simulink model "CAN_Model_v2"  (R2018b)
settings: Solver=VariableStepAuto  StartTime=0.0  StopTime=20  RelTol=1e-3
libraries: simulink_extras x1
settings Model: Creator=Emiliano  LastModifiedBy=Emiliano

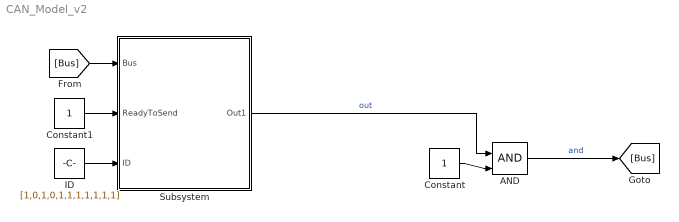
== system CAN_Model_v2 ==
  AND : Logic  IconShape=distinctive  AllPortsSameDT=off  OutDataTypeStr=boolean
  Constant : Constant  SampleTime=0.2
  Constant1 : Constant
  ID : Constant  Value=[1,0,1,0,1,1,1,1,1,1,1]
  Subsystem : Subsystem
  wires:
  Subsystem/1(Out1) -> AND/1  "out"
  Constant/1 -> AND/2
  AND/1 -> [Bus]  "and"
  [Bus] -> Subsystem/1(Bus)
  Constant1/1 -> Subsystem/2("ReadyToSend ")
  ID/1 -> Subsystem/3(ID)

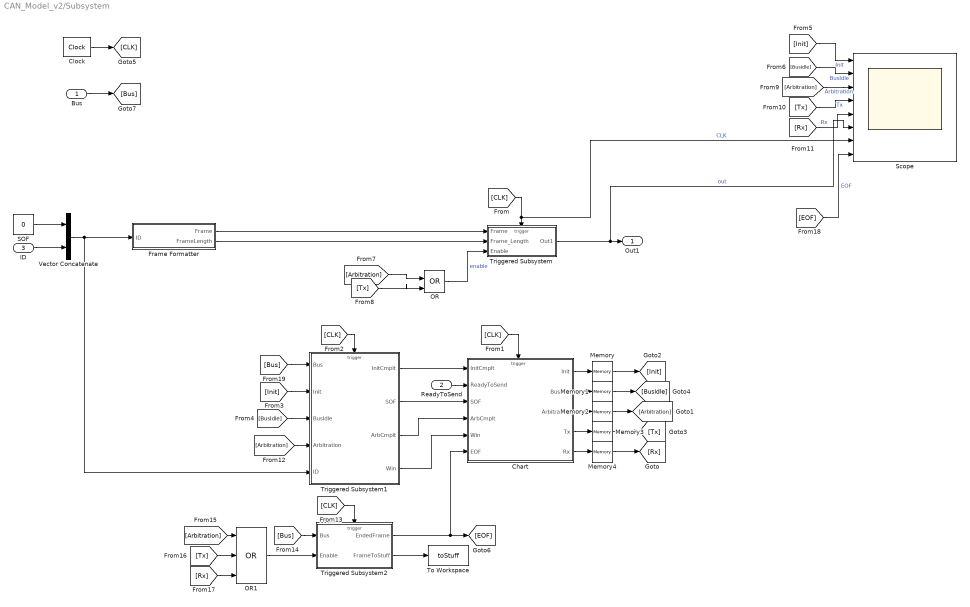
== system CAN_Model_v2/Subsystem ==
  Bus : Inport
  "ReadyToSend " : Inport  Port=2
  ID : Inport  Port=3
  Chart : Stateflow chart  TreatAsAtomicUnit=on
  Clock : simulink_extras/Flip Flops/Clock  period=0.2
  Frame Formatter : Subsystem
  Memory{,1..4} (5 alike) : Memory
  OR : Logic  Operator=OR  IconShape=distinctive  AllPortsSameDT=off  OutDataTypeStr=boolean
  OR1 : Logic  Operator=OR  Inputs=3  IconShape=distinctive  AllPortsSameDT=off  OutDataTypeStr=boolean
  SOF : Constant  Value=0
  Scope : Scope  NumInputPorts=8
  To Workspace : ToWorkspace  VariableName=toStuff  SaveFormat=Timeseries  SampleTime=-1
  Triggered Subsystem : Subsystem  TreatAsAtomicUnit=on
  Triggered Subsystem1 : Subsystem  TreatAsAtomicUnit=on
  Triggered Subsystem2 : Subsystem  TreatAsAtomicUnit=on
  Vector Concatenate : Concatenate
  Out1 : Outport
  wires:
  [CLK] -> Chart/Trigger
  [Arbitration] -> OR/1
  [Tx] -> OR/2
  OR/1 -> Triggered Subsystem/3(Enable)  "enable"
  Chart/5(" Rx") -> Memory4/1
  Chart/3(" Arbitration") -> Memory2/1
  Chart/1(" Init") -> Memory/1
  Chart/4(" Tx") -> Memory3/1
  Chart/2(" BusIdle") -> Memory1/1
  Clock/1 -> [CLK]
  [CLK] -> Scope/7, Triggered Subsystem/Trigger  "CLK"
  [CLK] -> Triggered Subsystem1/Trigger
  Triggered Subsystem1/1(InitCmplt) -> Chart/1(InitCmplt)
  [Init] -> Triggered Subsystem1/2(Init)
  "ReadyToSend "/1 -> Chart/2(ReadyToSend)
  [BusIdle] -> Triggered Subsystem1/3(BusIdle)
  Triggered Subsystem1/2(SOF) -> Chart/3(SOF)
  Triggered Subsystem1/4(Win) -> Chart/5(Win)
  Triggered Subsystem1/3("ArbCmplt ") -> Chart/4(ArbCmplt)
  [Init] -> Scope/1  "Init"
  [BusIdle] -> Scope/2  "BusIdle"
  [Arbitration] -> Scope/3  "Arbitration"
  [Tx] -> Scope/4  "Tx"
  [Rx] -> Scope/5  "Rx"
  Memory/1 -> [Init]
  Memory1/1 -> [BusIdle]
  Memory2/1 -> [Arbitration]
  Memory3/1 -> [Tx]
  Memory4/1 -> [Rx]
  Triggered Subsystem/1(Out1) -> Scope/6, Out1/1  "out"
  ID/1 -> Vector Concatenate/2
  [Arbitration] -> Triggered Subsystem1/4(Arbitration)
  [CLK] -> Triggered Subsystem2/Trigger
  [Bus] -> Triggered Subsystem2/1(Bus)
  OR1/1 -> Triggered Subsystem2/2(Enable)
  [Arbitration] -> OR1/1
  [Tx] -> OR1/2
  [Rx] -> OR1/3
  Triggered Subsystem2/1(EndedFrame) -> [EOF], Chart/6(EOF)
  Triggered Subsystem2/2(FrameToStuff) -> To Workspace/1
  [EOF] -> Scope/8  "EOF"
  Bus/1 -> [Bus]
  [Bus] -> Triggered Subsystem1/1(Bus)
  SOF/1 -> Vector Concatenate/1
  Vector Concatenate/1 -> Triggered Subsystem1/5(ID), Frame Formatter/1(ID)
  Frame Formatter/1(Frame) -> Triggered Subsystem/1("Frame ")
  Frame Formatter/2("FrameLength ") -> Triggered Subsystem/2(Frame_Length)

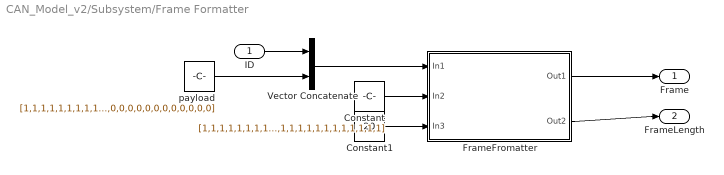
== system CAN_Model_v2/Subsystem/Frame Formatter ==
  ID : Inport
  Constant : Constant  Value=[1,1,1,1,1,1,1,1,1,1,1,1,1,1,1,1,1,1,1,1]
  Constant1 : Constant  Value=20
  FrameFromatter : Subsystem
  Vector Concatenate : Concatenate
  "payload " : Constant  Value=[1,1,1,1,1,1,1,1,1,1,1,1,1,1,1,1,1,1,1,0,0,0,0,0,0,0,0,0,0,0,0,0,0,0,0,0]
  Frame : Outport
  "FrameLength " : Outport  Port=2
  wires:
  ID/1 -> Vector Concatenate/1
  "payload "/1 -> Vector Concatenate/2
  Vector Concatenate/1 -> FrameFromatter/1(In1)
  Constant/1 -> FrameFromatter/2(In2)
  Constant1/1 -> FrameFromatter/3(In3)
  FrameFromatter/1(Out1) -> Frame/1
  FrameFromatter/2(Out2) -> "FrameLength "/1

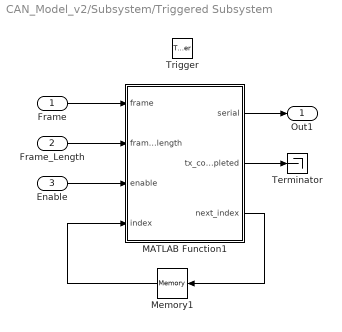
== system CAN_Model_v2/Subsystem/Triggered Subsystem ==
  "Frame " : Inport
  Frame_Length : Inport  Port=2
  Enable : Inport  Port=3
  Trigger : TriggerPort  VariantControl=Variant
  MATLAB Function1 : MATLAB Function  TreatAsAtomicUnit=on
  Memory1 : Memory  InitialCondition=1  InheritSampleTime=on
  Terminator : Terminator
  Out1 : Outport
  wires:
  Memory1/1 -> MATLAB Function1/4(index)
  MATLAB Function1/1(serial) -> Out1/1
  MATLAB Function1/3(next_index) -> Memory1/1
  MATLAB Function1/2(tx_completed) -> Terminator/1
  Enable/1 -> MATLAB Function1/3(enable)
  "Frame "/1 -> MATLAB Function1/1(frame)
  Frame_Length/1 -> MATLAB Function1/2(frame_length)

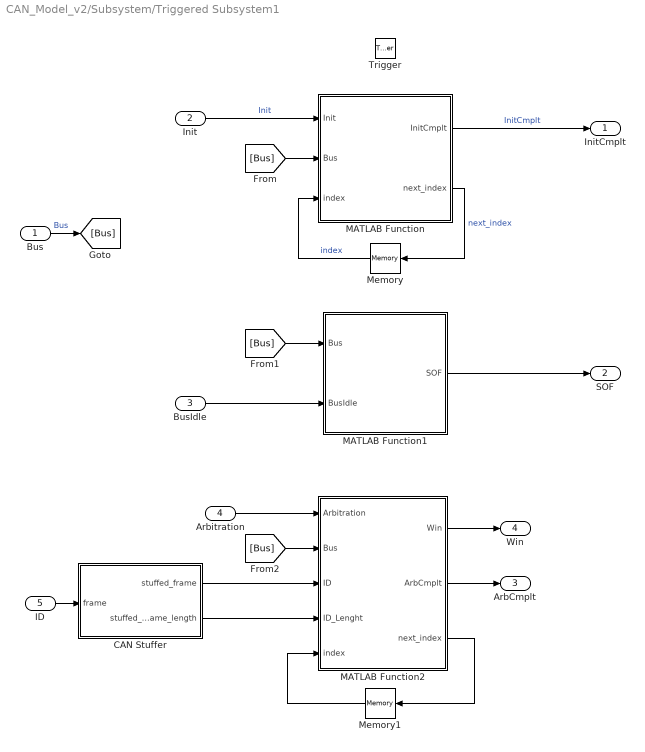
== system CAN_Model_v2/Subsystem/Triggered Subsystem1 ==
  Bus : Inport
  Init : Inport  Port=2
  BusIdle : Inport  Port=3
  Arbitration : Inport  Port=4
  ID : Inport  Port=5
  Trigger : TriggerPort  VariantControl=Variant
  CAN Stuffer : MATLAB Function  TreatAsAtomicUnit=on
  MATLAB Function : MATLAB Function  TreatAsAtomicUnit=on
  MATLAB Function1 : MATLAB Function  TreatAsAtomicUnit=on
  MATLAB Function2 : MATLAB Function  TreatAsAtomicUnit=on
  Memory : Memory  InheritSampleTime=on
  Memory1 : Memory  InitialCondition=1  InheritSampleTime=on
  InitCmplt : Outport
  SOF : Outport  Port=2
  "ArbCmplt " : Outport  Port=3
  Win : Outport  Port=4
  wires:
  MATLAB Function/2(next_index) -> Memory/1  "next_index"
  Memory/1 -> MATLAB Function/3(index)  "index"
  MATLAB Function/1(InitCmplt) -> InitCmplt/1  "InitCmplt"
  MATLAB Function1/1(SOF) -> SOF/1
  Init/1 -> MATLAB Function/1(Init)  "Init"
  BusIdle/1 -> MATLAB Function1/2(BusIdle)
  Arbitration/1 -> MATLAB Function2/1(Arbitration)
  Bus/1 -> [Bus]  "Bus"
  [Bus] -> MATLAB Function/2(Bus)
  [Bus] -> MATLAB Function1/1(Bus)
  [Bus] -> MATLAB Function2/2(Bus)
  MATLAB Function2/3(next_index) -> Memory1/1
  Memory1/1 -> MATLAB Function2/5(index)
  MATLAB Function2/1(Win) -> Win/1
  MATLAB Function2/2(ArbCmplt) -> "ArbCmplt "/1
  ID/1 -> CAN Stuffer/1(frame)
  CAN Stuffer/1(stuffed_frame) -> MATLAB Function2/3(ID)
  CAN Stuffer/2(stuffed_frame_length) -> MATLAB Function2/4(ID_Lenght)

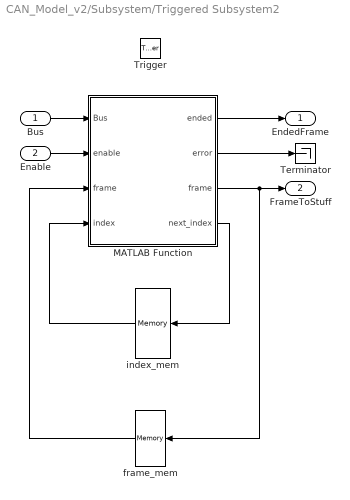
== system CAN_Model_v2/Subsystem/Triggered Subsystem2 ==
  Bus : Inport
  Enable : Inport  Port=2
  Trigger : TriggerPort  VariantControl=Variant
  MATLAB Function : MATLAB Function  TreatAsAtomicUnit=on
  Terminator : Terminator
  frame_mem : Memory  InitialCondition=[0,0,0,0,0,0,0,0,0,0,0,0,0,0,0,0,0,0,0,0,0,0,0,0,0,0,0,0,0,0,0,0,0,0,0,0,0,0,0,0,0,0,0,0,0,0,0,0,0,0,0,0,0,0,0,0,0,0,0,0,0,0,0,0,0,0,0,0,0,0,0,0,0,0,0,0,0,0,0,0,0,0,0,0,0,0,0,0,0,0,0,0,0,0,0,0,0,0,0,0,0,0,0,0,0,0,0,0,0,0,0,0,0,0,0,0,0,0,0,0,0,0,0,0,0,0,0,0,0,0,0,0,0,0,0]  InheritSampleTime=on
  index_mem : Memory  InitialCondition=1  InheritSampleTime=on
  EndedFrame : Outport
  FrameToStuff : Outport  Port=2
  wires:
  Enable/1 -> MATLAB Function/2(enable)
  Bus/1 -> MATLAB Function/1(Bus)
  MATLAB Function/4(next_index) -> index_mem/1
  frame_mem/1 -> MATLAB Function/3("frame ")
  MATLAB Function/1(ended) -> EndedFrame/1
  MATLAB Function/3(frame) -> frame_mem/1, FrameToStuff/1
  index_mem/1 -> MATLAB Function/4(index)
  MATLAB Function/2(error) -> Terminator/1

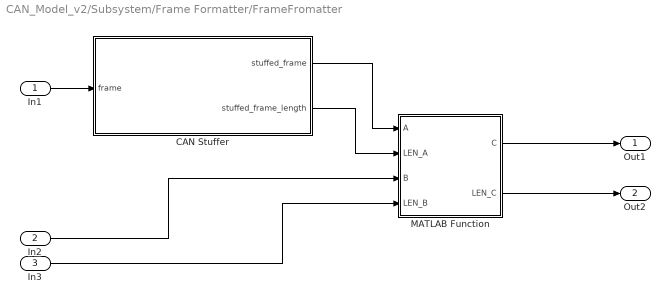
== system CAN_Model_v2/Subsystem/Frame Formatter/FrameFromatter ==
  In1 : Inport
  In2 : Inport  Port=2
  In3 : Inport  Port=3
  CAN Stuffer : MATLAB Function  TreatAsAtomicUnit=on
  MATLAB Function : MATLAB Function  TreatAsAtomicUnit=on
  Out1 : Outport
  Out2 : Outport  Port=2
  wires:
  MATLAB Function/2(LEN_C) -> Out2/1
  In1/1 -> CAN Stuffer/1(frame)
  CAN Stuffer/2(stuffed_frame_length) -> MATLAB Function/2(LEN_A)
  MATLAB Function/1(C) -> Out1/1
  In3/1 -> MATLAB Function/4(LEN_B)
  CAN Stuffer/1(stuffed_frame) -> MATLAB Function/1(A)
  In2/1 -> MATLAB Function/3(B)

== matlab function CAN_Model_v2/Subsystem/Triggered Subsystem1/MATLAB Function ==
  data: Init input; InitCmplt output; Bus input; index input; next_index output
function [InitCmplt, next_index] = BusIdleSensing(Init, Bus, index)

InitCmplt = 0;

if Init == 1
    if Bus == 1
        if index < 10 %Number of one to wait for EOF (after 11 ones)
            next_index = index + 1;
        else
            next_index = 0;
            InitCmplt = 1;
        end
    else
        next_index = 0;
    end
else
   next_index = 0;
end

end

== matlab function CAN_Model_v2/Subsystem/Triggered Subsystem/MATLAB Function1 ==
  data: frame input; frame_length input; enable input; serial output; tx_completed output; index input; next_index output
function [serial,  tx_completed ,next_index]  = fcn(frame, frame_length, enable, index)

if enable == 1
    if index > frame_length
        serial = 1;
        tx_completed = 1;
        next_index = 1;
    else
        serial = frame(index);
        next_index = index + 1;
        tx_completed = 0;
    end
else
    tx_completed = 0;
    serial = 1;
    next_index = 1;
end

end

== stateflow chart CAN_Model_v2/Subsystem/Chart ==
  settings: sampleTime=0.2  executeAtInitialization=1
  state Init
  state Rx
  state BusIdle
  state Arbitration
  state Tx
  Init -> Init [order 2] : [InitCmplt == 0]
  (default) -> Init
  Init -> BusIdle [order 1] : [InitCmplt == 1]
  Rx -> Rx [order 2] : [EOF == 0]
  BusIdle -> Rx [order 2] : [ReadyToSend == 0 && SOF == 1]
  Rx -> BusIdle [order 1] : [EOF == 1]
  BusIdle -> BusIdle [order 3] : [ReadyToSend == 0 && SOF == 0]
  Arbitration -> Rx [order 1] : [ArbCmplt ==1 && Win == 0]
  Tx -> BusIdle [order 2] : [EOF == 1]
  BusIdle -> Arbitration [order 1] : [ReadyToSend > 0]
  Arbitration -> Tx [order 2] : [ArbCmplt ==1 && Win == 1]
  Arbitration -> Arbitration [order 3] : [ArbCmplt == 0]
  Tx -> Tx [order 1] : [EOF == 0]
  data: Init output boolean; BusIdle output boolean; Arbitration output boolean; Tx output boolean; Rx output boolean; InitCmplt input; ReadyToSend input; SOF input; ArbCmplt input; Win input; EOF input
  events: Start input FALLING_EDGE_EVENT

== matlab function CAN_Model_v2/Subsystem/Triggered Subsystem1/MATLAB Function1 ==
  data: Bus input; SOF output; BusIdle input
function SOF = SOF_Detection(Bus, BusIdle)

if BusIdle == 1 %Checks the current state of the FSM
    if Bus == 0
        SOF = 1; %SOF Detected, the flag goes to One!
    else
        SOF = 0;    
    end
else
    SOF = 0;
end

end

== matlab function CAN_Model_v2/Subsystem/Triggered Subsystem1/MATLAB Function2 ==
  data: Win output; ArbCmplt output; Arbitration input; Bus input; ID input; ID_Lenght input; next_index output; index input
function [Win, ArbCmplt, next_index] = arbitration(Arbitration, Bus, ID, ID_Lenght, index)

ArbCmplt = 0;
Win = 0;
next_index = 1;

if Arbitration == 1
    if index <= ID_Lenght
        if ID(index) == Bus
            next_index = index + 1;
        else
            Win = 0;
            ArbCmplt = 1;
        end
    else
        next_index = 1;
        Win = 1;
        ArbCmplt = 1;
    end    
    
else next_index = 1;
    
end
end

== matlab function CAN_Model_v2/Subsystem/Triggered Subsystem1/CAN Stuffer ==
  data: frame input; stuffed_frame output; stuffed_frame_length output
function [stuffed_frame, stuffed_frame_length] = CANstuffer(frame)

NumOfZeros = 0;
NumOfOnes = 0;
NumOfStuffedBits = 0;

stuffed_frame = zeros(135,1);

for i = 1 : length(frame)
    if frame(i) == 0
        NumOfZeros = NumOfZeros + 1;
        NumOfOnes = 0;
    else
        NumOfOnes = NumOfOnes + 1;
        NumOfZeros = 0;
    end
    
    if NumOfZeros == 5
        NumOfZeros = 0;
        NumOfOnes = NumOfOnes + 1;
        
        %Appending the stuffed ONE
        stuffed_frame(i + NumOfStuffedBits) = frame(i);
        NumOfStuffedBits = NumOfStuffedBits + 1;
        stuffed_frame(i + NumOfStuffedBits) = 1;
        
    elseif NumOfOnes == 5
        NumOfOnes = 0;
        NumOfZeros = NumOfZeros + 1;
        
        %Appending the stuffed ZERO
        stuffed_frame(i + NumOfStuffedBits) = frame(i);
        NumOfStuffedBits = NumOfStuffedBits + 1;
        stuffed_frame(i + NumOfStuffedBits) = 0;
        
    else
        stuffed_frame(i + NumOfStuffedBits) = frame(i); 
    end
end
stuffed_frame_length = length(frame) + NumOfStuffedBits;
end

== matlab function CAN_Model_v2/Subsystem/Triggered Subsystem2/MATLAB Function ==
  data: ended output; error output; Bus input; enable input; frame output; frame input; index input; next_index output
%riempio il frame a partire da 135 (la sua lunghezza) per avere già gli elementi
%in ordine giusto (ma con degli zeri in più all'inizio)
function [ended, error, frame, next_index] = readBus(Bus, enable, frame, index)
ended=0;
error=0;
consecutive_ones=1;
consecutive_zeros=1;
next_index=1;
if enable==1
    
    if index<=135 %praticamente sempre
        
        frame(index)=Bus;
        next_index=index+1;
        
        for i = 1 : index-1
            if frame(i)==frame(i+1)
                if frame(i)==1
                    consecutive_ones=consecutive_ones+1;
                end
                if frame(i)==0
                    consecutive_zeros=consecutive_zeros+1;
                end
            end
            if frame(i)~=frame(i+1)
                consecutive_ones=1;
                consecutive_zeros=1;
            end

            if consecutive_ones==11
                ended=1;
                break;
            end
            if consecutive_zeros==7
                error=1;
                break;
            end
        end
        if ended==1 || error==1
            next_index=1;
        end
    else %non arrivo mai qui perché resetto l'indice già quando checkEOF==1 o ==2
        next_index=1; 
    end
    
end

end

== matlab function CAN_Model_v2/Subsystem/Frame Formatter/FrameFromatter/CAN Stuffer ==
  data: stuffed_frame output; stuffed_frame_length output; frame input
function [stuffed_frame, stuffed_frame_length] = CANstuffer(frame)

NumOfZeros = 0;
NumOfOnes = 0;
NumOfStuffedBits = 0;

stuffed_frame = zeros(135,1);

for i = 1 : length(frame)
    if frame(i) == 0
        NumOfZeros = NumOfZeros + 1;
        NumOfOnes = 0;
    else
        NumOfOnes = NumOfOnes + 1;
        NumOfZeros = 0;
    end
    
    if NumOfZeros == 5
        NumOfZeros = 0;
        NumOfOnes = NumOfOnes + 1;
        
        %Appending the stuffed ONE
        stuffed_frame(i + NumOfStuffedBits) = frame(i);
        NumOfStuffedBits = NumOfStuffedBits + 1;
        stuffed_frame(i + NumOfStuffedBits) = 1;
        
    elseif NumOfOnes == 5
        NumOfOnes = 0;
        NumOfZeros = NumOfZeros + 1;
        
        %Appending the stuffed ZERO
        stuffed_frame(i + NumOfStuffedBits) = frame(i);
        NumOfStuffedBits = NumOfStuffedBits + 1;
        stuffed_frame(i + NumOfStuffedBits) = 0;
        
    else
        stuffed_frame(i + NumOfStuffedBits) = frame(i); 
    end
end
stuffed_frame_length = length(frame) + NumOfStuffedBits;
end

== matlab function CAN_Model_v2/Subsystem/Frame Formatter/FrameFromatter/MATLAB Function ==
  data: A input; C output; LEN_A input; B input; LEN_B input; LEN_C output
function [C, LEN_C] = vectorAppend(A, LEN_A, B, LEN_B)

C = zeros(135,1);

for i = 1 : LEN_A
    C(i) = A(i);
end

for i = 1 : LEN_B
    C(LEN_A + i) = B(i);
end

LEN_C = LEN_A + LEN_B;
end
